simulink subsystem "mode_DDD"  (R2022a)
settings: Solver=VariableStepAuto  StartTime=0.0  StopTime=10.0  RelTol=1e-3
settings Model: Creator=bkfre  LastModifiedBy=bkfre

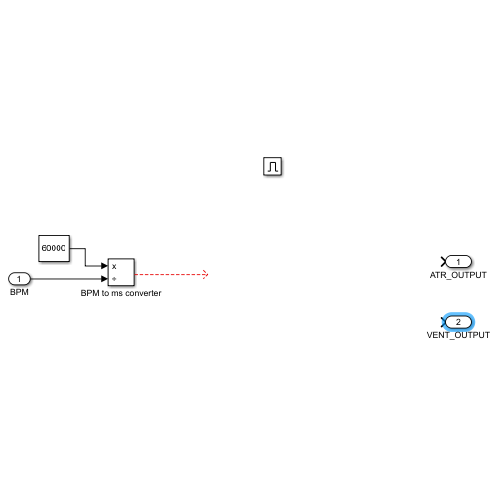
[thumbnail: Simulink's stored preview of the top-level diagram]
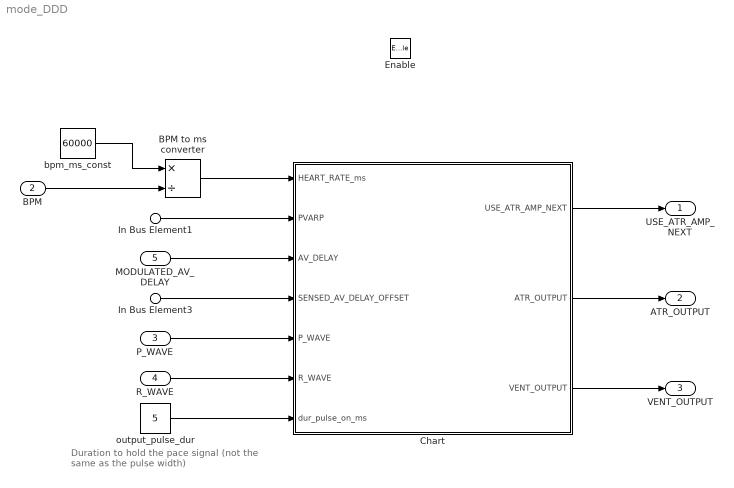
== system mode_DDD ==
  note: Duration to hold the pace signal (not the same as the pulse width)
  In Bus Element3 : Inport  PortName=BusGEN  Element=SENSED_AV_DELAY_OFFSET
  In Bus Element1 : Inport  PortName=BusGEN  Element=PVARP
  BPM : Inport  Port=2  OutDataTypeStr=double
  P_WAVE : Inport  Port=3
  R_WAVE : Inport  Port=4
  MODULATED_AV_DELAY : Inport  Port=5
  Enable : EnablePort
  BPM to ms converter : Product  Inputs=*/
  Chart : Stateflow chart  TreatAsAtomicUnit=on
      settings: PortSchema="{\"entries\":[{\"content\":{\"sides\":[{\"content\":{\"connectorIds\":[\"In1\",\"In2\",\"In3\",\"In7\",\"In4\",\"In5\",\"In6\"]},\"type\":\"ConnectorPlacement.EquallySpacedRectSide\",\"uuid\":\"56d1cac8-684f-45e6-a424-2234b0a4238e\"},{\"content\":{\"connectorIds\":[\"Out1\",\"Out2\",\"Out3\"],\"side\":\"RIGHT\"},\"type\":\"ConnectorPlacement.EquallySpacedRectSide\",\"uuid\":\"3f39bb9a-ffe3-4a99-90c1-38eb9ee50982\"},{\"content\":{\"connectorIds\":[],\"side\":\"TOP\"},\"type\":\"ConnectorPlacement.EquallySpacedRectSide\",\"uuid\":\"77d7a949-a54f-4f62-b3ae-491fde96a01d\"}]},\"type\":\"ConnectorPlacement.EquallySpacedConnector\",\"uuid\":\"873f3e9d-fdc0-4596-93d0-d0fa80b2dd62\"}],\"packageUris\":[\"http://schema.mathworks.com/mf0/Connector/R2020b\"],\"version\":\"1.0\"}"
  bpm_ms_const : Constant  Value=60000
  output_pulse_dur : Constant  Value=5
  USE_ATR_AMP_NEXT : Outport  OutDataTypeStr=boolean
  ATR_OUTPUT : Outport  Port=2
  VENT_OUTPUT : Outport  Port=3
  wires:
  In Bus Element3/1 -> Chart/7(SENSED_AV_DELAY_OFFSET)
  bpm_ms_const/1 -> BPM to ms converter/1
  BPM/1 -> BPM to ms converter/2
  BPM to ms converter/1 -> Chart/1(HEART_RATE_ms)
  Chart/3(VENT_OUTPUT) -> VENT_OUTPUT/1
  Chart/2(ATR_OUTPUT) -> ATR_OUTPUT/1
  Chart/1(USE_ATR_AMP_NEXT) -> USE_ATR_AMP_NEXT/1
  In Bus Element1/1 -> Chart/2(PVARP)
  MODULATED_AV_DELAY/1 -> Chart/3(AV_DELAY)
  P_WAVE/1 -> Chart/4(P_WAVE)
  R_WAVE/1 -> Chart/5(R_WAVE)
  output_pulse_dur/1 -> Chart/6(dur_pulse_on_ms)

== stateflow chart mode_DDD/Chart ==
  state ATR_ALERT
    entry:
    USE_ATR_AMP_NEXT = true;
    fix_timing = 0;
  state ATR_REFRACTORY
    entry:
    VENT_OUTPUT = 0;
  state ATR_PACE
    entry:
    ATR_OUTPUT = 1;
    fix_timing = dur_pulse_on_ms;
  state VENT_PACE
    entry:
    VENT_OUTPUT = 1;
    fix_timing = dur_pulse_on_ms;
  state VENT_ALERT
    entry:
    ATR_OUTPUT = 0;
    USE_ATR_AMP_NEXT = false;
  (default) -> ATR_REFRACTORY
  ATR_REFRACTORY -> ATR_ALERT : after(PVARP - fix_timing - offset, msec)
  ATR_ALERT -> ATR_PACE [order 2] : after(HEART_RATE_ms - AV_DELAY - PVARP,msec)
  VENT_PACE -> ATR_REFRACTORY : after(dur_pulse_on_ms,msec)
  VENT_ALERT -> ATR_REFRACTORY [order 1] : [R_WAVE]{offset = 0;}
  ATR_ALERT -> VENT_ALERT [order 1] : [P_WAVE]{
      | offset = SENSED_AV_DELAY_OFFSET;}
  ATR_PACE -> VENT_ALERT : after(dur_pulse_on_ms,msec){offset = 0;}
  VENT_ALERT -> VENT_PACE [order 2] : after(AV_DELAY - fix_timing + offset,msec)
  data: HEART_RATE_ms input; USE_ATR_AMP_NEXT output boolean; PVARP input; AV_DELAY input; P_WAVE input; R_WAVE input; ATR_OUTPUT output; VENT_OUTPUT output; dur_pulse_on_ms input; fix_timing local =0; SENSED_AV_DELAY_OFFSET input; offset local =0
